simulink model "tach"  (R2014a)
settings: Solver=FixedStepDiscrete  StartTime=0.0  StopTime=15  FixedStep=.001  RelTol=1e-3
libraries: embdlinuxlib x1, dspswit3 x1, dspsigops x1
settings Model: SimulationMode=external  ExtModeTrigDuration=100  Creator=Becky  LastModifiedBy=reck2
settings OptimizationCC: OptimizeModelRefInitCode=on  LifeSpan=1
settings DebuggingCC: UnderspecifiedInitializationDetection=Classic  SolverPrmCheckMsg=none
settings HardwareCC: ProdLargestAtomicInteger=Long  ProdLargestAtomicFloat=Double  ProdEndianess=LittleEndian  ProdHWDeviceType=ARM Compatible->ARM Cortex
settings RTWCC: SystemTargetFile=realtime.tlc  GenerateMakefile=off  TemplateMakefile=realtime.tmf  Description=Run on Target Hardware  RTWVerbose=off  ProcessScript=realtime_make_rtw_hook
settings STFCustomTargetCC: TargetLibSuffix=.a  GenerateSampleERTMain=on  ConcurrentExecutionCompliant=off  GeneratePreprocessorConditionals=Use local settings  ERTCustomFileBanners=on  SupportNonInlinedSFcns=off  SupportVariableSizeSignals=on  MATLABClassNameForMDSCustomization=Simulink.SoftwareTarget.ERTCustomization  GRTInterface=off  SystemTargetFile=realtime.tlc
settings ERTTargetCC: CombineOutputUpdateFcns=off  SupportContinuousTime=on  SupportVariableSizeSignals=on  ExtModeMexArgs='192.168.0.3' 0 17725  ERTSrcFileBannerTemplate=realtime_code_template.cgt  ERTHdrFileBannerTemplate=realtime_code_template.cgt  ERTDataSrcFileTemplate=realtime_code_template.cgt  ERTDataHdrFileTemplate=realtime_code_template.cgt  ERTCustomFileTemplate=realtime_file_process.tlc

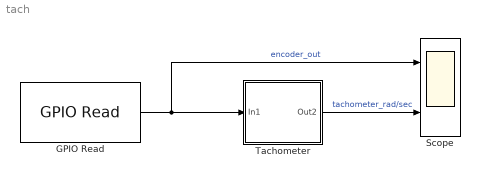
== system tach ==
  GPIO Read : embdlinuxlib/GPIO Read  board=Model B Rev2  gpio=22  internalResistor=Off  sampleTime=0.001  direction=Input  blockPlatform=Raspberry Pi
  Scope : Scope  NumInputPorts=2
      settings: TimeRange=15  YMin=-0.2~0  YMax=1.2~70
  Tachometer : Subsystem
  wires:
  GPIO Read/1 -> Scope/1, Tachometer/1(In1)  "encoder_out"
  Tachometer/1(Out2) -> Scope/2  "tachometer_rad/sec"

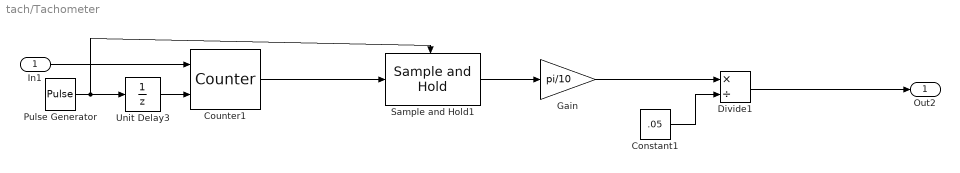
== system tach/Tachometer ==
  In1 : Inport
  Constant1 : Constant  Value=.05
  Counter1 : dspswit3/Counter  Direction=Up  CountEvent=Rising edge  CounterSize=User defined  MaxCount=256  InitialCount=0  Output=Count  HitValue=1  ResetInput=on  SamplesPerFrame=1  Ts=1  CntDtype=double  HitDtype=Logical
  Divide1 : Product  Inputs=*/
  Gain : Gain  Gain=pi/10
  Pulse Generator : DiscretePulseGenerator  PulseType=Time based  Period=.05  PulseWidth=10
  Sample and Hold1 : dspsigops/Sample and Hold  trig=Rising edge  initCond=1  latchinput=off
  Unit Delay3 : UnitDelay  SampleTime=-1
  Out2 : Outport
  wires:
  In1/1 -> Counter1/1
  Counter1/1 -> Sample and Hold1/1
  Constant1/1 -> Divide1/2
  Divide1/1 -> Out2/1
  Pulse Generator/1 -> Sample and Hold1/Trigger, Unit Delay3/1
  Gain/1 -> Divide1/1
  Unit Delay3/1 -> Counter1/2
  Sample and Hold1/1 -> Gain/1
